simulink model "FactorialUsingWhile"  (R2016b)
settings: Solver=FixedStepDiscrete  StartTime=0.0  StopTime=10.0  RelTol=1e-3
libraries: simulink x1
settings Model: Creator=Rasha  LastModifiedBy=Rasha
settings OptimizationCC: DefaultParameterBehavior=Inlined
settings DebuggingCC: ParameterTunabilityLossMsg=error
settings RTWCC: SystemTargetFile=ert.tlc  GenCodeOnly=on  TemplateMakefile=ert_default_tmf  Description=Embedded Coder  GenerateReport=on  IncludeHyperlinkInReport=on  LaunchReport=on  GenerateTraceInfo=on  GenerateTraceReport=on  GenerateTraceReportSl=on  GenerateTraceReportSf=on  GenerateTraceReportEml=on
settings CodeAppCC: ForceParamTrailComments=on  IgnoreCustomStorageClasses=off  OperatorAnnotations=on  SimulinkDataObjDesc=on  SFDataObjDesc=on  MATLABFcnDesc=on  InsertBlockDesc=on  MATLABSourceComments=on
settings ERTTargetCC: TargetLangStandard=C99 (ISO)  GenerateSampleERTMain=on  InlinedParameterPlacement=NonHierarchical  ERTCustomFileTemplate=example_file_process.tlc

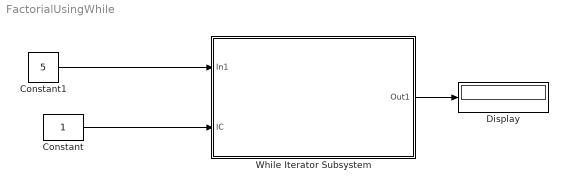
== system FactorialUsingWhile ==
  Constant : Constant
  Constant1 : Constant  Value=5
  Display : Display
  While Iterator Subsystem : Subsystem  TreatAsAtomicUnit=on
  wires:
  Constant/1 -> While Iterator Subsystem/2(IC)
  Constant1/1 -> While Iterator Subsystem/1(In1)
  While Iterator Subsystem/1(Out1) -> Display/1

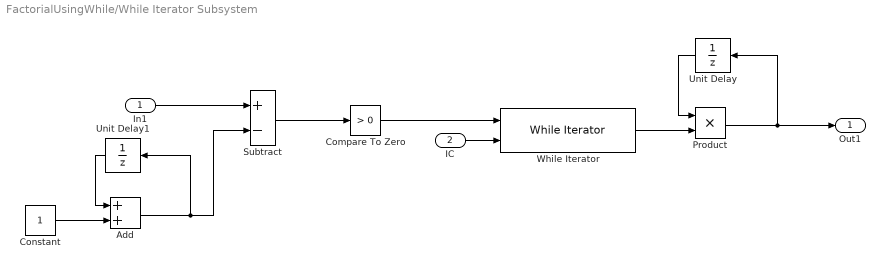
== system FactorialUsingWhile/While Iterator Subsystem ==
  In1 : Inport
  IC : Inport  Port=2
  Add : Sum
  Compare To Zero : simulink/Logic and Bit Operations/Compare To Zero  relop=>  OutDataTypeStr=boolean
  Constant : Constant
  Product : Product
  Subtract : Sum  Inputs=+-
  Unit Delay : UnitDelay  InitialCondition=1  SampleTime=-1
  Unit Delay1 : UnitDelay  SampleTime=-1
  While Iterator : WhileIterator  ShowIterationPort=on  OutputDataType=double
  Out1 : Outport
  wires:
  IC/1 -> While Iterator/2
  Compare To Zero/1 -> While Iterator/1
  While Iterator/1 -> Product/2
  Unit Delay/1 -> Product/1
  Product/1 -> Out1/1, Unit Delay/1
  Subtract/1 -> Compare To Zero/1
  In1/1 -> Subtract/1
  Add/1 -> Unit Delay1/1, Subtract/2
  Constant/1 -> Add/2
  Unit Delay1/1 -> Add/1
